simulink model "nsdynamic_Force2"  (R2021b)
settings: Solver=ode4  StartTime=0.0  StopTime=10.0  RelTol=1e-3
InitFcn:
  | initialization
undefined symbols (not defined in the file or in its folder): dynNS_Force2, trajectory
settings Model: Creator=AzamaoZ  LastModifiedBy=AzamaoZ

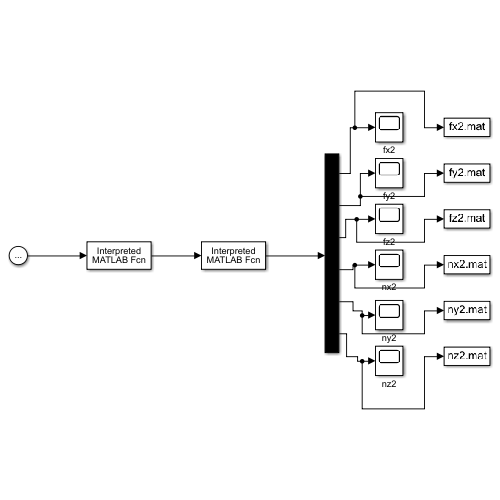
[thumbnail: Simulink's stored preview of the top-level diagram]
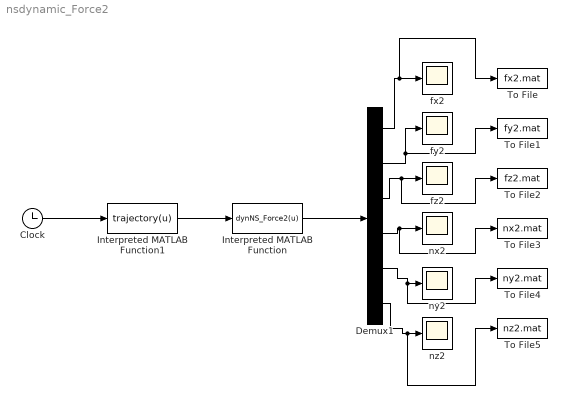
== system nsdynamic_Force2 ==
  Clock : Clock
  Demux1 : Demux  Outputs=6
  Interpreted MATLAB Function : MATLABFcn  MATLABFcn=dynNS_Force2(u)  OutputDimensions=6
  Interpreted MATLAB Function1 : MATLABFcn  MATLABFcn=trajectory(u)
  To File : ToFile  Filename=fx2.mat  MatrixName=fx2  SaveFormat=Timeseries
  To File1 : ToFile  Filename=fy2.mat  MatrixName=fy2  SaveFormat=Timeseries
  To File2 : ToFile  Filename=fz2.mat  MatrixName=fz2  SaveFormat=Timeseries
  To File3 : ToFile  Filename=nx2.mat  MatrixName=nx2  SaveFormat=Timeseries
  To File4 : ToFile  Filename=ny2.mat  MatrixName=ny2  SaveFormat=Timeseries
  To File5 : ToFile  Filename=nz2.mat  MatrixName=nz2  SaveFormat=Timeseries
  fx2 : Scope
  fy2 : Scope
  fz2 : Scope
  nx2 : Scope
  ny2 : Scope
  nz2 : Scope
  wires:
  Interpreted MATLAB Function/1 -> Demux1/1
  Clock/1 -> Interpreted MATLAB Function1/1
  Demux1/2 -> fy2/1, To File1/1
  Demux1/4 -> To File3/1, nx2/1
  Demux1/6 -> To File5/1, nz2/1
  Demux1/5 -> To File4/1, ny2/1
  Demux1/3 -> To File2/1, fz2/1
  Interpreted MATLAB Function1/1 -> Interpreted MATLAB Function/1
  Demux1/1 -> To File/1, fx2/1
